simulink subsystem "LED_Sensores"  (R2023b)
settings: Solver=VariableStepAuto  StartTime=0.0  StopTime=10.0  RelTol=1e-3
libraries: simulink x3
settings Model: Creator=javie  LastModifiedBy=javie

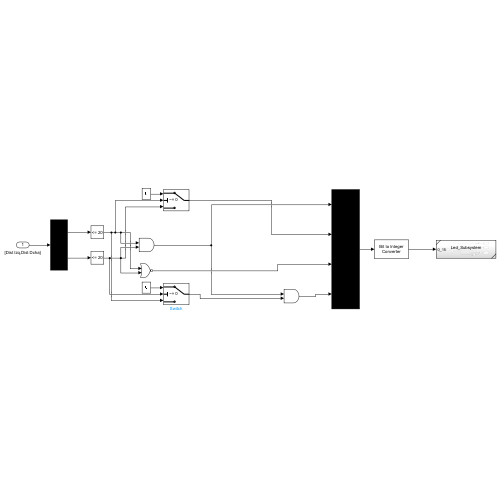
[thumbnail: Simulink's stored preview of the top-level diagram]
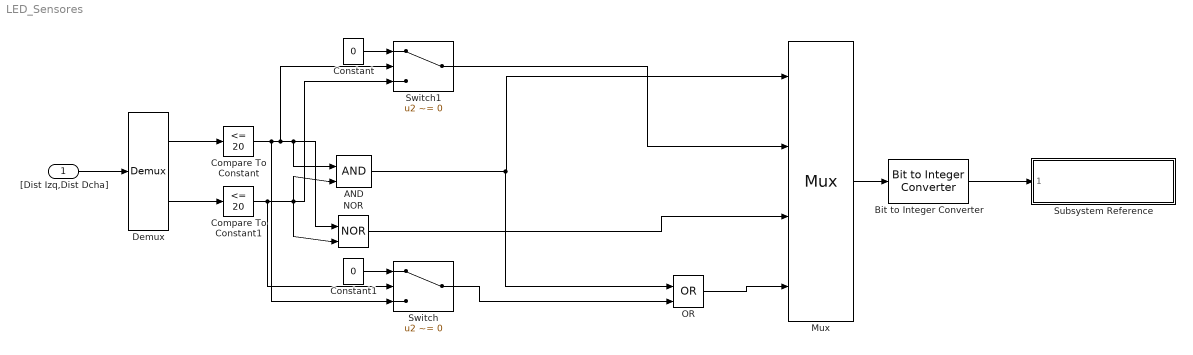
== system LED_Sensores ==
  "[Dist Izq,Dist Dcha]" : Inport
  AND : Logic  IconShape=distinctive  AllPortsSameDT=off  OutDataTypeStr=boolean
  Bit to Integer Converter : simulink/Logic and Bit Operations/Bit to Integer Converter  nbits=4  bitOrder=MSB first  signedOutputValues=Unsigned  outDtype=Inherit via internal rule  outDtypeSigned=Inherit via internal rule
  Compare To Constant : simulink/Logic and Bit Operations/Compare To Constant  relop=<=  const=20  OutDataTypeStr=boolean
  Compare To Constant1 : simulink/Logic and Bit Operations/Compare To Constant  relop=<=  const=20  OutDataTypeStr=boolean
  Constant : Constant  Value=0
  Constant1 : Constant  Value=0
  Demux : Demux  Outputs=2
  Mux : Mux
  NOR : Logic  Operator=NOR  IconShape=distinctive  AllPortsSameDT=off  OutDataTypeStr=boolean
  OR : Logic  Operator=OR  IconShape=distinctive  AllPortsSameDT=off  OutDataTypeStr=boolean
  Subsystem Reference : Subsystem  ReferencedSubsystem=Led_Subsystem
  Switch : Switch  Criteria=u2 ~= 0  OutDataTypeStr=boolean  SaturateOnIntegerOverflow=off  InputSameDT=off
  Switch1 : Switch  Criteria=u2 ~= 0  Threshold=20  OutDataTypeStr=boolean  SaturateOnIntegerOverflow=off  InputSameDT=off
  wires:
  Mux/1 -> Bit to Integer Converter/1
  Bit to Integer Converter/1 -> Subsystem Reference/1
  "[Dist Izq,Dist Dcha]"/1 -> Demux/1
  Demux/1 -> Compare To Constant/1
  Demux/2 -> Compare To Constant1/1
  NOR/1 -> Mux/3
  Compare To Constant/1 -> Switch/3, Switch1/2, AND/1, NOR/1
  Compare To Constant1/1 -> Switch/2, Switch1/3, AND/2, NOR/2
  AND/1 -> Mux/1, OR/1
  Switch1/1 -> Mux/2
  Constant/1 -> Switch1/1
  Switch/1 -> OR/2
  Constant1/1 -> Switch/1
  OR/1 -> Mux/4
